simulink model "Ident_2"  (Simulink 7.6)
settings: Solver=ode45  StartTime=0.0  StopTime=inf  RelTol=1e-3
libraries: opclib x5
settings Model: Creator=Administrator  LastModifiedBy=Administrator

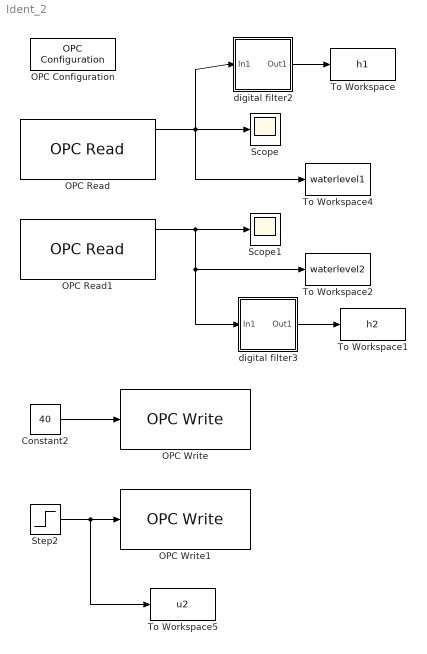
== system Ident_2 ==
  Constant2 : Constant  Value=40
  OPC Configuration : opclib/OPC Configuration  opcServers=localhost/OPCServer.WinCC/10  errMissingItems=Error  errReadWrite=Warn  errShutdown=Error  errRTViolation=Warn  rtEnable=on  speedup=1  showLatency=off  beingUsed=on
  OPC Read : opclib/OPC Read  serverHost=localhost  serverID=OPCServer.WinCC  itemIDs=shuiwei1  readMode=Synchronous (cache)  dataType=double  updateRate=0.5  showQual=on  showTS=on  tsMode=Seconds since start
  OPC Read1 : opclib/OPC Read  serverHost=localhost  serverID=OPCServer.WinCC  itemIDs=shuiwei2  readMode=Synchronous (cache)  dataType=double  updateRate=0.5  showQual=on  showTS=on  tsMode=Seconds since start
  OPC Write : opclib/OPC Write  serverHost=localhost  serverID=OPCServer.WinCC  itemIDs=beng1  writeMode=Synchronous  updateRate=0
  OPC Write1 : opclib/OPC Write  serverHost=localhost  serverID=OPCServer.WinCC  itemIDs=beng2  writeMode=Synchronous  updateRate=0
  Scope : Scope
      settings: TimeRange=500  YMin=10  YMax=11
  Scope1 : Scope
      settings: TimeRange=500  YMin=9  YMax=11
  Step2 : Step  Time=500  Before=40  After=50
  To Workspace : ToWorkspace  VariableName=h1  SampleTime=1  SaveFormat=Array
  To Workspace1 : ToWorkspace  VariableName=h2  SampleTime=1  SaveFormat=Array
  To Workspace2 : ToWorkspace  VariableName=waterlevel2  SampleTime=1  SaveFormat=Array
  To Workspace4 : ToWorkspace  VariableName=waterlevel1  SampleTime=1  SaveFormat=Array
  To Workspace5 : ToWorkspace  VariableName=u2  SampleTime=1  SaveFormat=Array
  digital filter2 : Subsystem
      mask Display: disp('filter')
  digital filter3 : Subsystem
      mask Display: disp('filter')
  wires:
  Constant2/1 -> OPC Write/1
  OPC Read/1 -> To Workspace4/1, Scope/1, digital filter2/1(In1)
  OPC Read1/1 -> Scope1/1, To Workspace2/1, digital filter3/1(In1)
  Step2/1 -> OPC Write1/1, To Workspace5/1
  digital filter3/1(Out1) -> To Workspace1/1
  digital filter2/1(Out1) -> To Workspace/1

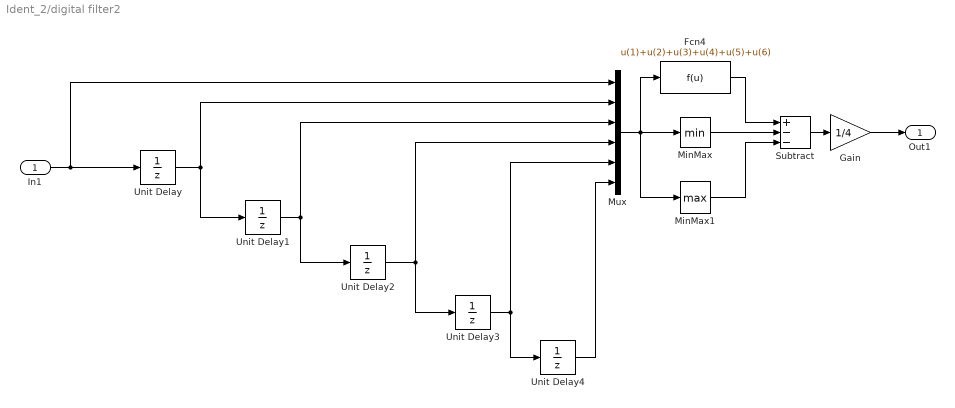
== system Ident_2/digital filter2 ==
  In1 : Inport
  Fcn4 : Fcn  Expr=u(1)+u(2)+u(3)+u(4)+u(5)+u(6)  SampleTime=0.5
  Gain : Gain  Gain=1/4
  MinMax : MinMax
  MinMax1 : MinMax  Function=max
  Mux : Mux  Inputs=6
  Subtract : Sum  Inputs=+--
  Unit Delay{,1..4} (5 alike) : UnitDelay  SampleTime=0.5
  Out1 : Outport
  wires:
  Gain/1 -> Out1/1
  Unit Delay4/1 -> Mux/6
  Subtract/1 -> Gain/1
  MinMax1/1 -> Subtract/3
  MinMax/1 -> Subtract/2
  Fcn4/1 -> Subtract/1
  Mux/1 -> MinMax1/1, MinMax/1, Fcn4/1
  Unit Delay3/1 -> Unit Delay4/1, Mux/5
  In1/1 -> Mux/1, Unit Delay/1
  Unit Delay2/1 -> Unit Delay3/1, Mux/4
  Unit Delay1/1 -> Unit Delay2/1, Mux/3
  Unit Delay/1 -> Unit Delay1/1, Mux/2

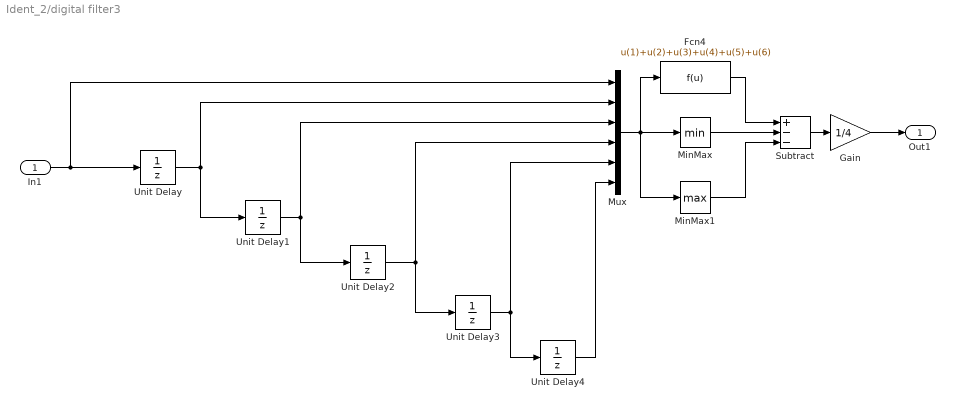
== system Ident_2/digital filter3 ==
  In1 : Inport
  Fcn4 : Fcn  Expr=u(1)+u(2)+u(3)+u(4)+u(5)+u(6)  SampleTime=0.5
  Gain : Gain  Gain=1/4
  MinMax : MinMax
  MinMax1 : MinMax  Function=max
  Mux : Mux  Inputs=6
  Subtract : Sum  Inputs=+--
  Unit Delay{,1..4} (5 alike) : UnitDelay  SampleTime=0.5
  Out1 : Outport
  wires:
  Unit Delay/1 -> Mux/2, Unit Delay1/1
  Unit Delay1/1 -> Mux/3, Unit Delay2/1
  Unit Delay2/1 -> Mux/4, Unit Delay3/1
  In1/1 -> Unit Delay/1, Mux/1
  Unit Delay3/1 -> Mux/5, Unit Delay4/1
  Mux/1 -> Fcn4/1, MinMax/1, MinMax1/1
  Fcn4/1 -> Subtract/1
  MinMax/1 -> Subtract/2
  MinMax1/1 -> Subtract/3
  Subtract/1 -> Gain/1
  Unit Delay4/1 -> Mux/6
  Gain/1 -> Out1/1
